simulink model "Tyre_Pac96_firstOrder"  (R2023b)
settings: Solver=ode4  StartTime=0.0  StopTime=200  FixedStep=0.001  RelTol=1e-3
values from neighbouring files (symbols this model uses):
  Af = 2.36    [Load_Params.m]
  batt_cap = 58e3    (= 58000)    [Load_Params.m]
  cog = .55    (= 0.55)    [Load_Params.m]
  Cx = .27    (= 0.27)    [Load_Params.m]
  eta_t = .9    (= 0.9)    [Load_Params.m]
  f0 = 0.009    [Load_Params.m]
  f2 = 6.5e-6    (= 6.5e-06)    [Load_Params.m]
  FZR_st = kerb_w*g*a/wheelbase    (= 8887.86)    [Load_Params.m]
  inertia = 1    [Load_Params.m]
  kerb_w = 1812    [Load_Params.m]
  mech_eff = .95    (= 0.95)    [Load_Params.m]
  Pacn = Pace'    [Load_Tyre_Data.m]
  peak_pw = 150e3    (= 150000)    [Load_Params.m]    (also in tractive_effort.m)
  rho = 1.2    [Load_Params.m]
  rpm_max = 16e3    (= 16000)    [Load_Params.m]
  tau_g = 10.5    [Load_Params.m]
  torque_max = 310    [Load_Params.m]    (also in tractive_effort.m)
  v_base = peak_pw/torque_max    (= 483.870967742)    [Load_Params.m]    (also in tractive_effort.m)
  velstart = 0.01    [Load_Params.m]
  wheel_radius = wheel_prof+rim_size    (= 0.5901)    [Load_Params.m]
  wheelbase = 2.77    [Load_Params.m]
undefined symbols (not defined in the file or in its folder): me, x0
libraries: simulink x1
settings Model: Creator=Nico  LastModifiedBy=edoardocavallotti
settings SolverCC: AlgebraicLoopSolver=TrustRegion
settings DataIOCC: LimitDataPoints=on  SaveFormat=Array  SignalLoggingSaveFormat=ModelDataLogs  ReturnWorkspaceOutputs=off  SignalLoggingName=sigsOut
settings OptimizationCC: BooleanDataType=off  InitFltsAndDblsToZero=on  LifeSpan=inf
settings DebuggingCC: SaveWithParameterizedLinksMsg=none  UnderspecifiedInitializationDetection=Classic  MergeDetectMultiDrivingBlocksExec=none  SignalResolutionControl=TryResolveAllWithWarning  MultiTaskDSMMsg=warning  MultiTaskCondExecSysMsg=none  FcnCallInpInsideContextMsg=warning  UnconnectedInputMsg=warning  UnconnectedOutputMsg=warning  UnconnectedLineMsg=warning  AllowSymbolicDim=off  SFUnexpectedBacktrackingDiag=warning  SFNoUnconditionalDefaultTransitionDiag=warning  SFExecutionAtInitializationDiag=none  ArithmeticOperatorsInVariantConditions=warning
settings HardwareCC: ProdBitPerPointer=32  ProdBitPerSizeT=32  ProdBitPerPtrDiffT=32  ProdLargestAtomicFloat=None  ProdIntDivRoundTo=Undefined  ProdEndianess=Unspecified  ProdWordSize=32  ProdHWDeviceType=32-bit Generic  TargetUnknown=on
settings ModelReferenceCC: EnableRefExpFcnMdlSchedulingChecks=on  PropagateSignalLabelsOutOfModel=off
settings SFSimCC: SimUseLocalCustomCode=off  SimParseCustomCode=off  CustomCodeUndefinedFunction=UseInterfaceOnly
settings RTWCC: RTWUseLocalCustomCode=off  DLArmComputeVersion=19.05
settings CodeAppCC: StateflowObjectComments=on
settings GRTTargetCC: TargetFcnLib=ansi_tfl_tmw.mat  TargetLangStandard=C89/C90 (ANSI)  CombineOutputUpdateFcns=off  GRTInterface=on
settings ConfigComp: CovMetricSettings=dw  CovSaveCumulativeToWorkspaceVar=on  CovSaveSingleToWorkspaceVar=on  CovExternalEMLEnable=off

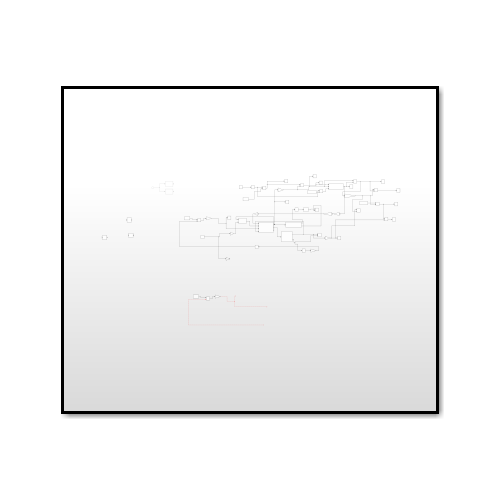
[thumbnail: Simulink's stored preview of the top-level diagram]
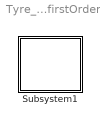
== system Tyre_Pac96_firstOrder ==
  Subsystem1 : Subsystem

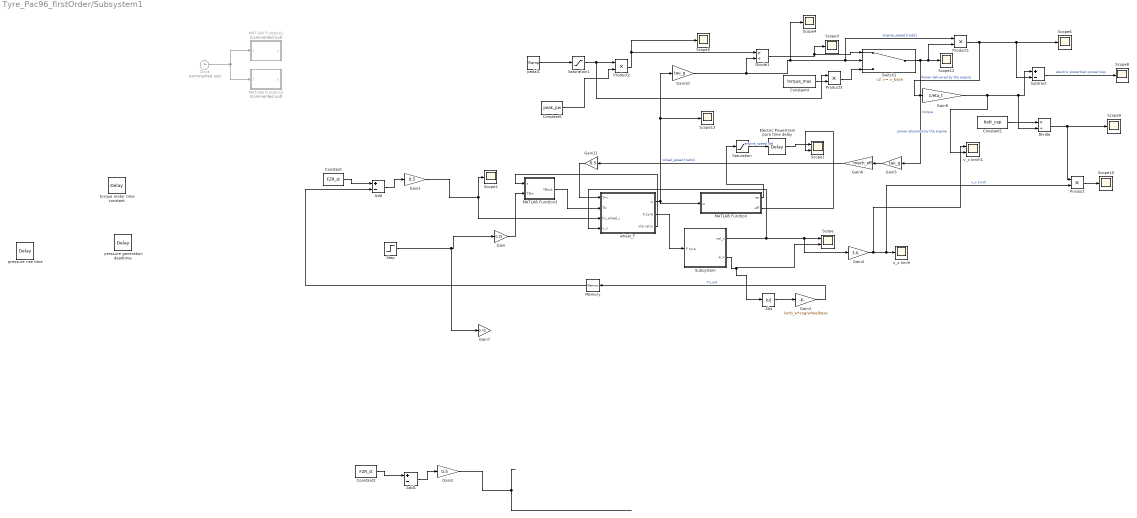
== system Tyre_Pac96_firstOrder/Subsystem1 ==
  "   torque motor time constant" : TransportDelay  DelayTime=0.05
  " pressure generation deadtime" : TransportDelay  DelayTime=0.02
  Abs : Abs  SaturateOnIntegerOverflow=off
  Add : Sum  Inputs=+-
  Add1 : Sum  Inputs=+-
  Clock : Clock  Commented=on
  Constant : Constant  Value=FZR_st
  Constant1 : Constant  Value=batt_cap
  Constant2 : Constant  Value=FZR_st
  Constant4 : Constant  Value=torque_max  VectorParams1D=off
  Constant5 : Constant  Value=peak_pw  VectorParams1D=off
  Divide : Product  Inputs=*/
  Divide1 : Product  Inputs=*/
  Electric Powertrain pure time delay : TransportDelay  DelayTime=0.02
  Gain : Gain  Gain=0.25
  Gain1 : Gain  Gain=0.5
  Gain10 : Gain  Gain=tau_g
  Gain11 : Gain  Gain=0.5
  Gain2 : Gain  Gain=0.5
  Gain3 : Gain  Gain=kerb_w*cog/wheelbase
  Gain4 : Gain  Gain=3.6
  Gain5 : Gain  Gain=tau_g
  Gain6 : Gain  Gain=mech_eff
  Gain7 : Gain  Gain=0.75
  Gain9 : Gain  Gain=1/eta_t
  MATLAB Function : MATLAB Function  TreatAsAtomicUnit=on
  MATLAB Function1 : MATLAB Function  Commented=on  TreatAsAtomicUnit=on
  MATLAB Function2 : MATLAB Function  Commented=on  TreatAsAtomicUnit=on
  MATLAB Function3 : MATLAB Function  TreatAsAtomicUnit=on
  Memory : Memory
  Product{,1..3} (4 alike) : Product
  Saturation : Saturate  UpperLimit=rpm_max  LowerLimit=0
  Saturation1 : Saturate  UpperLimit=0.08  LowerLimit=0
  Scope : Scope  NumInputPorts=2
  Scope1 : Scope  NumInputPorts=2
  Scope{2..6,8..10,12..13} (10 alike) : Scope
  Step : Step  Time=2  After=500  SampleTime=0
  Subsystem : Subsystem
  Subtract : Sum  Inputs=+-
  Switch1 : Switch  Threshold=v_base  SaturateOnIntegerOverflow=off  InputSameDT=off
  pedal1 : simulink/Sources/Ramp  slope=4  start=0  InitialOutput=0
  "pressure rise time " : TransportDelay  DelayTime=0.025
  v_x km/h : Scope
  v_x km/h1 : Scope  NumInputPorts=2
  wheel_F : Subsystem
  wires:
  wheel_F/2(F_tyre) -> Subsystem/1(F tyre)
  Subsystem/1(vel_x) -> wheel_F/4(v_x), Gain4/1, Scope/1
  Subsystem/2(a_x) -> Abs/1, Scope/2
  Gain1/1 -> Scope2/1, wheel_F/3(Fz_wheel_i)
  wheel_F/1(w) -> MATLAB Function/1(w), Scope13/1, Gain10/1  "wheel_speed [rad/s]"
  Constant/1 -> Add/1
  Add/1 -> Gain1/1
  Abs/1 -> Gain3/1
  Gain3/1 -> Memory/1  "Fz_w4"
  MATLAB Function/1(es) -> Saturation/1
  Saturation/1 -> Electric Powertrain pure time delay/1  "engine_speed_del"
  Electric Powertrain pure time delay/1 -> Scope1/1
  Memory/1 -> Add/2
  Step/1 -> Gain7/1, Gain/1
  MATLAB Function/2(eff) -> Scope1/2
  Gain2/1 -> ?
  Add1/1 -> Gain2/1
  Constant2/1 -> Add1/1
  ? -> Add1/2
  Gain4/1 -> v_x km/h1/1, Product/2, v_x km/h/1  "v_x km/h"
  Switch1/1 -> Product1/2, Scope12/1, Gain5/1  "torque"
  Constant4/1 -> Product3/2
  Constant5/1 -> Product2/2
  Saturation1/1 -> Product3/1, Product2/1
  pedal1/1 -> Saturation1/1
  Divide1/1 -> Scope3/1, Switch1/1
  Product2/1 -> Divide1/1, Scope5/1
  Gain10/1 -> Product1/1, Switch1/2, Scope4/1, Divide1/2  "engine_speed [rad/s]"
  Product3/1 -> Switch1/3
  Clock/1 -> MATLAB Function2/1(t), MATLAB Function1/1(t)
  Gain5/1 -> Gain6/1
  Gain6/1 -> Gain11/1
  Gain11/1 -> wheel_F/1(Tm)
  Product1/1 -> Gain9/1, Scope6/1, Subtract/2  "Power delivered by the engine"
  Gain9/1 -> v_x km/h1/2, Divide/2, Subtract/1  "power absorbed by the engine"
  Subtract/1 -> Scope8/1  "electric powertrain power loss"
  Constant1/1 -> Divide/1
  Divide/1 -> Product/1, Scope9/1
  Product/1 -> Scope10/1
  wheel_F/3(slip ratio) -> MATLAB Function3/1(s)
  MATLAB Function3/1(TBout) -> wheel_F/2(Tb)
  Gain/1 -> MATLAB Function3/2(TBin)

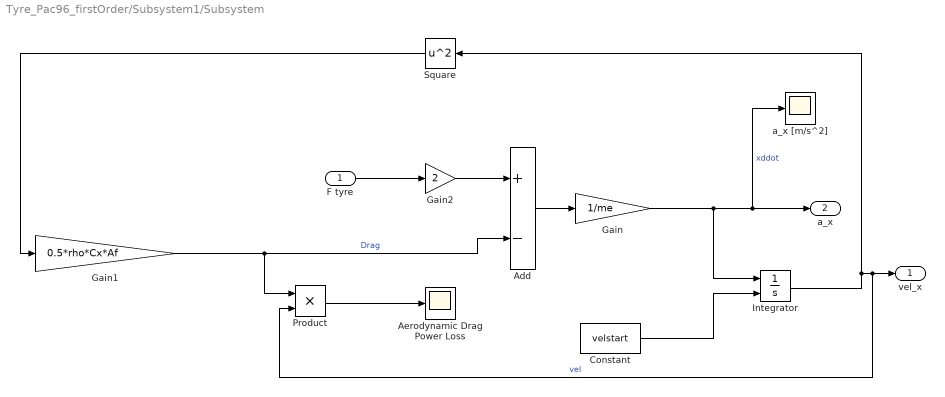
== system Tyre_Pac96_firstOrder/Subsystem1/Subsystem ==
  F tyre : Inport
  Add : Sum  Inputs=+-
  Aerodynamic Drag Power Loss : Scope
  Constant : Constant  Value=velstart
  Gain : Gain  Gain=1/me
  Gain1 : Gain  Gain=0.5*rho*Cx*Af
  Gain2 : Gain  Gain=2
  Integrator : Integrator  InitialConditionSource=external
  Product : Product
  Square : Math  Operator=square
  a_x [m/s^2] : Scope
  vel_x : Outport
  a_x : Outport  Port=2
  wires:
  Constant/1 -> Integrator/2
  Gain/1 -> Integrator/1, a_x [m/s^2]/1, a_x/1  "xddot"
  Integrator/1 -> Square/1, Product/2, vel_x/1  "vel"
  F tyre/1 -> Gain2/1
  Gain2/1 -> Add/1
  Gain1/1 -> Product/1, Add/2  "Drag"
  Square/1 -> Gain1/1
  Add/1 -> Gain/1
  Product/1 -> Aerodynamic Drag Power Loss/1

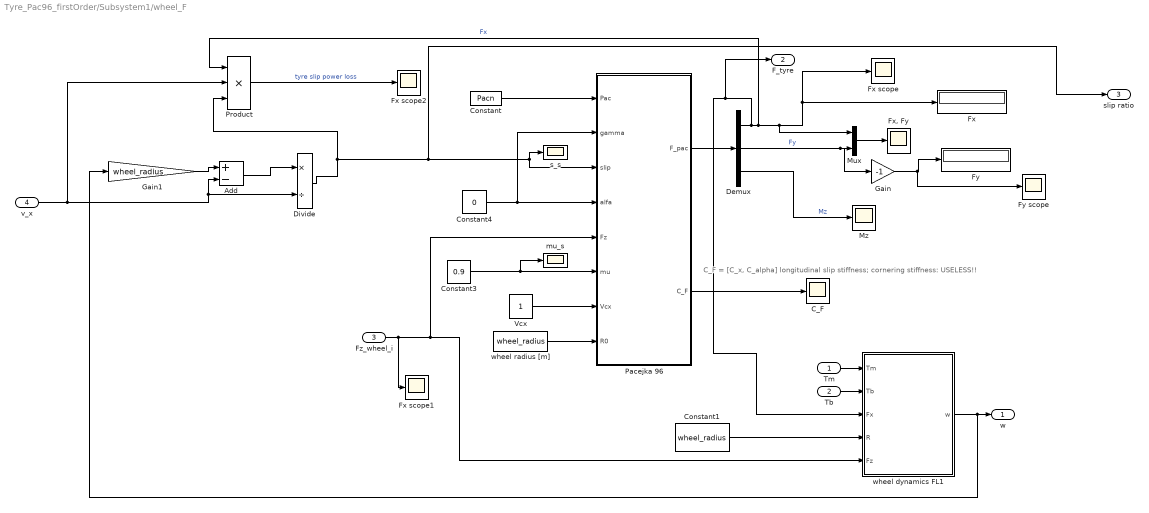
== system Tyre_Pac96_firstOrder/Subsystem1/wheel_F ==
  note: C_F = [C_x, C_alpha] longitudinal slip stiffness; cornering stiffness: USELESS!!
  Tm : Inport
  Tb : Inport  Port=2
  Fz_wheel_i : Inport  Port=3
  v_x : Inport  Port=4
  Add : Sum  Inputs=+-
  C_F : Scope
  Constant : Constant  Value=Pacn
  Constant1 : Constant  Value=wheel_radius
  Constant3 : Constant  Value=0.9
  Constant4 : Constant  Value=0
  Demux : Demux  Outputs=3
  Divide : Product  Inputs=*/
  Fx : Display
  Fx scope : Scope
  Fx scope1 : Scope
  Fx scope2 : Scope
  "Fx, Fy" : Scope
  Fy : Display
  Fy scope : Scope
  Gain : Gain  Gain=-1
  Gain1 : Gain  Gain=wheel_radius
  Mux : Mux  Inputs=2
  Mz : Scope
  Pacejka 96 : MATLAB Function  TreatAsAtomicUnit=on
  Product : Product  Inputs=3
  Vcx : Constant
  mu_s : Scope
  s_s : Scope
  wheel dynamics FL1 : Subsystem
  wheel radius [m] : Constant  Value=wheel_radius
  w : Outport
  F_tyre : Outport  Port=2
  slip ratio : Outport  Port=3
  wires:
  Tm/1 -> wheel dynamics FL1/1(Tm)
  wheel dynamics FL1/1(w) -> Gain1/1, w/1
  Constant1/1 -> wheel dynamics FL1/4(R)
  Constant/1 -> Pacejka 96/1(Pac)
  Divide/1 -> Product/3, slip ratio/1, Pacejka 96/3(slip), s_s/1
  Mux/1 -> "Fx, Fy"/1
  Vcx/1 -> Pacejka 96/7(Vcx)
  wheel radius [m]/1 -> Pacejka 96/8(R0)
  Demux/1 -> F_tyre/1, wheel dynamics FL1/3(Fx), Product/1, Mux/1, Fx/1, Fx scope/1  "Fx"
  Constant3/1 -> mu_s/1, Pacejka 96/6(mu)
  Pacejka 96/2(C_F) -> C_F/1
  Gain/1 -> Fy scope/1, Fy/1
  Demux/2 -> Gain/1, Mux/2  "Fy"
  Tb/1 -> wheel dynamics FL1/2(Tb)
  Pacejka 96/1(F_pac) -> Demux/1
  Demux/3 -> Mz/1  "Mz"
  Fz_wheel_i/1 -> Fx scope1/1, wheel dynamics FL1/5(Fz), Pacejka 96/5(Fz)
  Constant4/1 -> Pacejka 96/2(gamma), Pacejka 96/4(alfa)
  Gain1/1 -> Add/1
  Add/1 -> Divide/1
  v_x/1 -> Product/2, Add/2, Divide/2
  Product/1 -> Fx scope2/1  "tyre slip power loss"

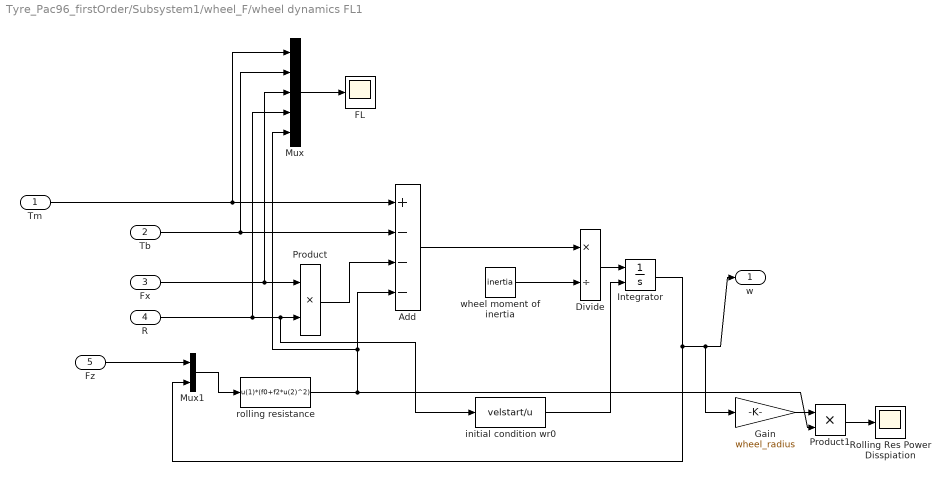
== system Tyre_Pac96_firstOrder/Subsystem1/wheel_F/wheel dynamics FL1 ==
  Tm : Inport
  Tb : Inport  Port=2
  Fx : Inport  Port=3
  R : Inport  Port=4
  Fz : Inport  Port=5
  Add : Sum  Inputs=+---
  Divide : Product  Inputs=*/
  FL : Scope
  Gain : Gain  Gain=wheel_radius
  Integrator : Integrator  InitialConditionSource=external  InitialCondition=x0
  Mux : Mux  Inputs=5
  Mux1 : Mux  Inputs=2
  Product : Product
  Product1 : Product
  Rolling Res Power Disspiation : Scope
  initial condition wr0 : MATLABFcn  MATLABFcn=velstart/u
  rolling resistance : MATLABFcn  MATLABFcn=u(1)*(f0+f2*u(2)^2)
  wheel moment of inertia : Constant  Value=inertia
  w : Outport
  wires:
  Tm/1 -> Mux/1, Add/1
  R/1 -> Mux/4, initial condition wr0/1, Product/2
  rolling resistance/1 -> Product1/2, Add/4, Mux/5
  Tb/1 -> Mux/2, Add/2
  Fx/1 -> Mux/3, Product/1
  Product/1 -> Add/3
  Mux/1 -> FL/1
  Add/1 -> Divide/1
  Divide/1 -> Integrator/1
  initial condition wr0/1 -> Integrator/2
  Mux1/1 -> rolling resistance/1
  wheel moment of inertia/1 -> Divide/2
  Integrator/1 -> Mux1/2, Gain/1, w/1
  Fz/1 -> Mux1/1
  Gain/1 -> Product1/1
  Product1/1 -> Rolling Res Power Disspiation/1

== matlab function Tyre_Pac96_firstOrder/Subsystem1/wheel_F/Pacejka 96 ==
  settings: fimath=|
      | fimath(...
      | 'RoundMode', 'floor',...
      | 'OverflowMode', 'wrap',...
      | 'ProductMode', 'KeepLSB', 'ProductWordLength', 32,...
      | 'SumMode', 'KeepLSB', 'SumWordLength', 32,...
      | 'CastBeforeSum', false)
  data: Pac input; gamma input; slip input; alfa input; Fz input; F_pac output; mu input; Vcx input; C_F output; R0 input
function [F_pac,C_F] = fcn(Pac,gamma,slip,alfa,Fz,mu,Vcx,R0)
% function for computing forces Fx, Fy and self-aligning torque Mz

% Pac   -> model structure with coeff. Pacejka 96
% slip  -> slip ratio [-] (-1:1)
% alfa  -> slip angle [rad]
% gamma -> camber [rad]
% Vcx,y velocity components of tire contact point C

% Structure building: Pacejka model coefficients
Pa_FZ0_ = Pac(1);
Pa_LFZ0 = Pac(2);
Pa_LmuV = Pac(3);
Pa_LKXK = Pac(4);
Pa_LKYA = Pac(5);
Pa_LCX_ = Pac(6);
Pa_LCY_ = Pac(7);
Pa_LEX_ = Pac(8);
Pa_LEY_ = Pac(9);
Pa_LHX_ = Pac(10);
Pa_LHY_ = Pac(11);
Pa_LVX_ = Pac(12);
Pa_LVY_ = Pac(13);
Pa_LKYG = Pac(14);
Pa_LKZG = Pac(15);
Pa_LT__ = Pac(16);
Pa_MR__ = Pac(17);
Pa_LXA_ = Pac(18);
Pa_LYK_ = Pac(19);
Pa_LVYK = Pac(20);
Pa_LS__ = Pac(21);
Pa_LCZ_ = Pac(22);
Pa_LMX_ = Pac(23);
Pa_LMY_ = Pac(24);
Pa_PCX1 = Pac(25);
Pa_PDX1 = Pac(26);
Pa_PDX2 = Pac(27);
Pa_PEX1 = Pac(28);
Pa_PEX2 = Pac(29);
Pa_PEX3 = Pac(30);
Pa_PEX4 = Pac(31);
Pa_PKX1 = Pac(32);
Pa_PKX2 = Pac(33);
Pa_PKX3 = Pac(34);
Pa_PHX1 = Pac(35);
Pa_PHX2 = Pac(36);
Pa_PVX1 = Pac(37);
Pa_PVX2 = Pac(38);
Pa_RBX1 = Pac(39);
Pa_RBX2 = Pac(40);
Pa_RCX1 = Pac(41);
Pa_RHX1 = Pac(42);
Pa_RTX1 = Pac(43);
Pa_RTX2 = Pac(44);
Pa_RTX3 = Pac(45);
Pa_QSX1 = Pac(46);
Pa_QSX2 = Pac(47);
Pa_QSX3 = Pac(48);
Pa_PCY1 = Pac(49);
Pa_PDY1 = Pac(50);
Pa_PDY2 = Pac(51);
Pa_PDY3 = Pac(52);
Pa_PEY1 = Pac(53);
Pa_PEY2 = Pac(54);
Pa_PEY3 = Pac(55);
Pa_PEY4 = Pac(56);
Pa_PKY1 = Pac(57);
Pa_PKY2 = Pac(58);
Pa_PKY3 = Pac(59);
Pa_PHY1 = Pac(60);
Pa_PHY2 = Pac(61);
Pa_PHY3 = Pac(62);
Pa_PVY1 = Pac(63);
Pa_PVY2 = Pac(64);
Pa_PVY3 = Pac(65);
Pa_PVY4 = Pac(66);
Pa_RBY1 = Pac(67);
Pa_RBY2 = Pac(68);
Pa_RBY3 = Pac(69);
Pa_RCY1 = Pac(70);
Pa_RHY1 = Pac(71);
Pa_RVY1 = Pac(72);
Pa_RVY2 = Pac(73);
Pa_RVY3 = Pac(74);
Pa_RVY4 = Pac(75);
Pa_RVY5 = Pac(76);
Pa_RVY6 = Pac(77);
Pa_PTY1 = Pac(78);
Pa_PTY2 = Pac(79);
Pa_QSY1 = Pac(80);
Pa_QSY2 = Pac(81);
Pa_QBZ1 = Pac(82);
Pa_QBZ2 = Pac(83);
Pa_QBZ3 = Pac(84);
Pa_QBZ4 = Pac(85);
Pa_QBZ5 = Pac(86);
Pa_QBZ6 = Pac(87);
Pa_QBZ9 = Pac(88);
Pa_QBZZ = Pac(89);
Pa_QCZ1 = Pac(90);
Pa_QDZ1 = Pac(91);
Pa_QDZ2 = Pac(92);
Pa_QDZ3 = Pac(93);
Pa_QDZ4 = Pac(94);
Pa_QDZ6 = Pac(95);
Pa_QDZ7 = Pac(96);
Pa_QDZ8 = Pac(97);
Pa_QDZ9 = Pac(98);
Pa_QEZ1 = Pac(99);
Pa_QEZ2 = Pac(100);
Pa_QEZ3 = Pac(101);
Pa_QEZ4 = Pac(102);
Pa_QEZ5 = Pac(103);
Pa_QHZ1 = Pac(104);
Pa_QHZ2 = Pac(105);
Pa_QHZ3 = Pac(106);
Pa_QHZ4 = Pac(107);
Pa_SSZ1 = Pac(108);
Pa_SSZ2 = Pac(109);
Pa_SSZ3 = Pac(110);
Pa_SSZ4 = Pac(111);
Pa_QTZ1 = Pac(112);

% Costants
epsi = 0.01;
eps_V = 0.1;
csi_0=1;
csi_4=1;
Amu = 10;
Pa_LmuX = mu;
Pa_LmuY = mu;

%-------------------------------- Fx pure slip ---------------------------
Cx = Pa_PCX1*Pa_LCX_;
dfz = (Fz-Pa_LFZ0*Pa_FZ0_)/(Pa_LFZ0*Pa_FZ0_);
mux = Pa_LmuX * (Pa_PDX1 + Pa_PDX2 * dfz);
Dx = mux*Fz; %*csi_1, con csi_1=1
%Shx = (Pa_PHX1+Pa_PHX2*dfz)*Pa_LHX_;
Shx = 0;
Kx = slip + Shx;
Ex = (Pa_PEX1+Pa_PEX2*dfz+Pa_PEX3*dfz^2)*(1-Pa_PEX4*sign(Kx))*Pa_LEX_;
if Ex>1 Et=1; end
Kxk = Fz*(Pa_PKX1+Pa_PKX2*dfz)*exp(Pa_PKX3*dfz)*Pa_LKXK;
Bx = Kxk/(Cx*Dx+epsi);
lam_mux  = Pa_LmuX*Amu/(1+(Amu-1)*Pa_LmuX);
SVx = Fz*(Pa_PVX1+Pa_PVX2*dfz)*(abs(Vcx)/(abs(Vcx)+eps_V))*Pa_LVX_*lam_mux; %*csi_1, con csi_1=1

% logitudinal slip stiffness (Fx slope in the origin)
C_Fk = Bx*Cx*Dx;

% longitudinal force
Fx0 = Dx*sin(Cx*atan(Bx*Kx-Ex*(Bx*Kx-atan(Bx*Kx)))) + SVx;

%---------------------------- Fy pure side slip --------------------------
seg=sign(Vcx);
if seg==0 seg=1; end
alfa_star = tan(alfa)*seg;
gam_star = sin(gamma);
Shy = (Pa_PHY1+Pa_PHY2*dfz)*Pa_LHY_+Pa_PHY3*gam_star*Pa_LKYG*csi_0+csi_4-1;
alfa_y = alfa_star + Shy;
Cy = Pa_PCY1*Pa_LCY_;
muy = Pa_LmuY*(Pa_PDY1+Pa_PDY2*dfz)*(1-Pa_PDY3*gam_star^2);
Dy = muy*Fz; %*csi_2, con csi_2=1
Ey = (Pa_PEY1+Pa_PEY2*dfz)*(1-(Pa_PEY3+Pa_PEY4*gam_star)*sign(alfa_y))*Pa_LEY_;
if Ey>1 Ey=1; end
Kya0 = Pa_PKY1*Pa_LFZ0*Pa_FZ0_*sin(2*atan(Fz/(Pa_PKY2*Pa_LFZ0*Pa_FZ0_)))*Pa_LKYA;
Kya = Kya0*(1-Pa_PKY3*gam_star^2); %*csi_3, con csi_3=1
By = Kya/(Cy*Dy+epsi);
lam_muy = Pa_LmuY*Amu/(1+(Amu-1)*Pa_LmuY);
SVy = Fz*((Pa_PVY1+Pa_PVY2*dfz)*Pa_LVY_+(Pa_PVY3+Pa_PVY4*dfz)*gam_star*Pa_LKYG )*lam_muy; %*csi_2, con csi_2=1
Kyg0 = (Pa_PHY3*Kya0+Fz*(Pa_PVY3+Pa_PVY4*dfz))*Pa_LKYG;

% cornering stiffness (Fy slope in the origin)
C_Fa = By*Cy*Dy;

% lateral force
Fy0 = Dy*sin(Cy*atan(By*alfa_y-Ey*(By*alfa_y-atan(By*alfa_y)))) + SVy;

% --------------------- Fx combined slip ------------------------------
Shxa = Pa_RHX1;
%Exa = Pa_REX1+Pa_REX2*dfz; NON esiste Pa.REX1 ne' Pa.REX2
Exa = 0;
Cxa = Pa_RCX1;
Bxa = Pa_RBX1*cos(atan(Pa_RBX2*slip))*Pa_LXA_;
alfaS = alfa_star+Shxa;
Gxa0 = cos(Cxa*atan(Bxa*Shxa-Exa*(Bxa*Shxa-atan(Bxa*Shxa))));
Gxa = cos(Cxa*atan(Bxa*alfaS-Exa*(Bxa*alfaS-atan(Bxa*alfaS))))/Gxa0;
Fx = Fx0*Gxa;

% ---------------------- Fy combined slip ------------------------------
Dvyk = muy*Fz*(Pa_RVY1+Pa_RVY2*dfz+Pa_RVY3*gam_star)*cos(atan(Pa_RVY4*alfa_star));%*csi_2, con csi_2=1
Svyk = Dvyk*sin(Pa_RVY5*atan(Pa_RVY6*slip));
Shyk = Pa_RHY1; %+Pa.RHY2*dfz; NON esiste Pa.RHY2
Cyk = Pa_RCY1;
Byk = Pa_RBY1*cos(atan(Pa_RBY2*(alfa_star-Pa_RBY3)))*Pa_LYK_;
%Eyk = Pa_REY1+Pa_REY2*dfz; NON esiste Pa.REY1 ne' Pa.REY2
Eyk = 0;
ks = slip+Shyk;
Gyk0 = cos(Cyk*atan(Byk*Shyk-Eyk*(Byk*Shyk-atan(Byk*Shyk))));
Gyk = cos(Cyk*atan(Byk*ks-Eyk*(Byk*ks-atan(Byk*ks))))/Gyk0;
Fy = Fy0*Gyk+Svyk;

% --------------------- Mz pure side slip  ---------------------------
Shf = Shy+SVy/Kya;
alfa_r = alfa_star+Shf;
Br = (Pa_QBZ9/Pa_LmuY+Pa_QBZZ*By*Cy); %*csi_6, con csi_6=1
%%% Pa_QBZZ e' in realta' QBZ10 scritto cosi' x ragioni di spazio
Cr = 1; %*csi_7, con csi_7=1
Dr = Fz*R0*((Pa_QDZ6+Pa_QDZ7*dfz)+(Pa_QDZ8+Pa_QDZ9*dfz)*gam_star)*cos(alfa)*Pa_LmuY*seg; %+csi_8-1, con csi_8=1
Mzr0 = Dr*cos(Cr*atan(Br*alfa_r));
Sht = Pa_QHZ1+Pa_QHZ2*dfz+(Pa_QHZ3+Pa_QHZ4*dfz)*gam_star;
alfa_t = alfa_star+Sht;
Bt = (Pa_QBZ1+Pa_QBZ2*dfz+Pa_QBZ3*dfz^2)*(1+Pa_QBZ5*abs(gam_star)+Pa_QBZ6*gam_star^2)*Pa_LKYA/Pa_LmuY;
if Bt<0 Bt=0; end
Ct = Pa_QCZ1;
Dt0 = Fz*R0/(Pa_LFZ0*Pa_FZ0_)*(Pa_QDZ1+Pa_QDZ2*dfz)*seg;
Dt = Dt0*(1+Pa_QDZ3*abs(gam_star)+Pa_QDZ4*gam_star^2); %*csi_5, con csi_5=1
Et = (Pa_QEZ1+Pa_QEZ2*dfz+Pa_QEZ3*dfz^2)*(1+(Pa_QEZ4+Pa_QEZ5*gam_star)*2/pi*atan(Bt*Ct*alfa_t));
if Et>1 Et=1; end
t0 = Dt*cos(Ct*atan(Bt*alfa_t - Et*(Bt*alfa_t-atan(Bt*alfa_t))))*cos(alfa);
Mz0 = -t0*Fy;
Kza0 = Dt0*Kya0;
%Kzg0 = Fz*R0*(Pa_QDZ8+Pa_QDZ9*dfz)-Dt0*Kyg0;

% aligning torque
Mz = Mz0 + Mzr0;

% ------------------------ Mz Combined -----------------------------
eps_k = 0; % 
lambda_s = Pa_LS__ ;
Fz0p = Pa_LFZ0*Pa_FZ0_;
K_yap = Kya + eps_k;
alfa_req = sqrt(alfa_r^2+(Kxk/K_yap)^2*slip^2)*sign(alfa_r);
alfa_teq = sqrt(alfa_t^2+(Kxk/K_yap)^2*slip^2)*sign(alfa_t);
s = R0*(Pa_SSZ1 + Pa_SSZ2*(Fy/Fz0p) + (Pa_SSZ3+Pa_SSZ4*dfz)*gam_star)*lambda_s;
Mzr = Dr*cos(Cr*atan(Br*alfa_req));
Fyp = Fy-Svyk; 
t = Dt*cos(Ct*atan(Bt*alfa_teq - Et*(Bt*alfa_teq-atan(Bt*alfa_teq))))*cos(alfa);
Mzp = -t*Fyp;
% aligning torque
Mz = Mzp + Mzr + s*Fx;
%%%%%%%%%%%%%%%%%%%%%%%

% Check that Fz is positive
if Fz <= 0
    Fx = 0;
    Fy = 0;
    Mz = 0;
end

% Output
F_pac = [Fx; Fy; Mz];
C_F = [C_Fk; C_Fa];

== matlab function Tyre_Pac96_firstOrder/Subsystem1/MATLAB Function ==
  data: w input; es output; eff output
function [es, eff] = tractive_effort(w)
% v vel veicolo
% vel ang ruota


eta_t = 0.9;
tau_g = 10.5; % gear ratio

es = w*tau_g;


peak_pw = 150e3; 
torque_max = 310;


v_base = peak_pw/torque_max; % vel ang motore

if es > v_base
    eff = peak_pw/es;
else
    eff = torque_max;
end

end

== matlab function Tyre_Pac96_firstOrder/Subsystem1/MATLAB Function1 ==
  data: t input; y output
function y = fcn(t)

if t < 10
    y = 0;
else
    y = 10;
end

== matlab function Tyre_Pac96_firstOrder/Subsystem1/MATLAB Function2 ==
  data: t input; y output
function y = fcn(t)

y = t;

== matlab function Tyre_Pac96_firstOrder/Subsystem1/MATLAB Function3 ==
  data: s input; TBout output; TBin input
function TBout = ABS(s, TBin)

if s>0.12
    TBout = TBin/2;
else
    TBout = TBin;
end
